simulink model "first"  (R2023a)
settings: Solver=FixedStepAuto  StartTime=0.0  StopTime=100  FixedStep=0.0001  RelTol=1e-3
settings Model: Creator=evdokiiagalkina  LastModifiedBy=evdokiiagalkina

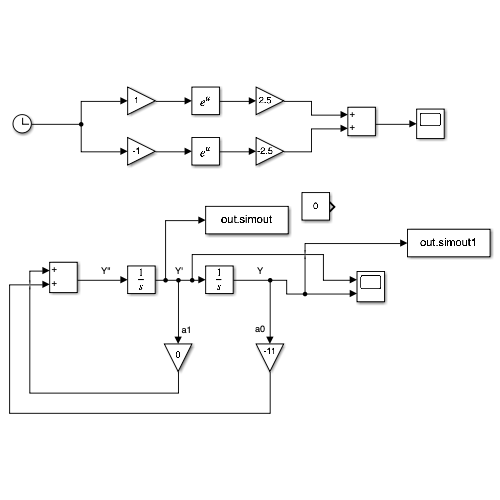
[thumbnail: Simulink's stored preview of the top-level diagram]
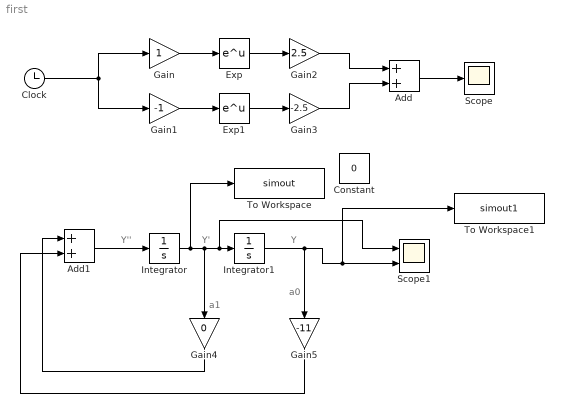
== system first ==
  note: a0
  note: a1
  note: Y
  note: Y'
  note: Y''
  Add : Sum
  Add1 : Sum
  Clock : Clock
  Constant : Constant  Value=0  SampleTime=-1
  Exp : Math  OutputSignalType=real
  Exp1 : Math  OutputSignalType=real
  Gain : Gain
  Gain1 : Gain  Gain=-1
  Gain2 : Gain  Gain=2.5
  Gain3 : Gain  Gain=-2.5
  Gain4 : Gain  Gain=0
  Gain5 : Gain  Gain=-11
  Integrator : Integrator  InitialCondition=10
  Integrator1 : Integrator  InitialCondition=5
  Scope : Scope
  Scope1 : Scope  NumInputPorts=2
  To Workspace : ToWorkspace  VariableName=simout  SaveFormat=Timeseries  SampleTime=-1
  To Workspace1 : ToWorkspace  VariableName=simout1  SaveFormat=Timeseries  SampleTime=-1
  wires:
  Gain/1 -> Exp/1
  Gain1/1 -> Exp1/1
  Add/1 -> Scope/1
  Clock/1 -> Gain1/1, Gain/1
  Exp1/1 -> Gain3/1
  Exp/1 -> Gain2/1
  Gain2/1 -> Add/1
  Gain3/1 -> Add/2
  Add1/1 -> Integrator/1
  Gain5/1 -> Add1/2
  Gain4/1 -> Add1/1
  Integrator1/1 -> To Workspace1/1, Scope1/2, Gain5/1
  Integrator/1 -> To Workspace/1, Gain4/1, Scope1/1, Integrator1/1
